simulink model "uklad2"  (R2023a)
settings: Solver=VariableStepAuto  StartTime=0.0  StopTime=200  RelTol=1e-3
undefined symbols (not defined in the file): kr, T, Tp
settings Model: Creator=jpawl  LastModifiedBy=jpawl

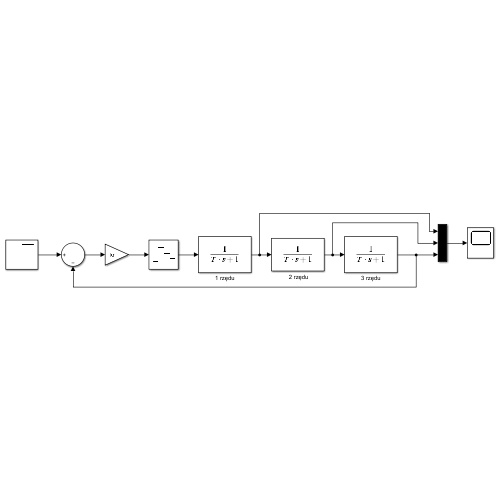
[thumbnail: Simulink's stored preview of the top-level diagram]
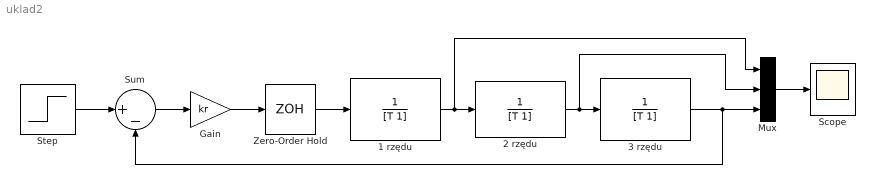
== system uklad2 ==
  " 2 rzędu" : TransferFcn  Denominator=[T 1]
  1 rzędu : TransferFcn  Denominator=[T 1]
  3 rzędu : TransferFcn  Denominator=[T 1]
  Gain : Gain  Gain=kr
  Mux : Mux  Inputs=3
  Scope : Scope
  Step : Step  SampleTime=Tp
  Sum : Sum  Inputs=|+-
  Zero-Order Hold : ZeroOrderHold  SampleTime=Tp
  wires:
  Step/1 -> Sum/1
  Sum/1 -> Gain/1
  Gain/1 -> Zero-Order Hold/1
  " 2 rzędu"/1 -> Mux/2, 3 rzędu/1
  1 rzędu/1 -> Mux/1, " 2 rzędu"/1
  Zero-Order Hold/1 -> 1 rzędu/1
  3 rzędu/1 -> Mux/3, Sum/2
  Mux/1 -> Scope/1
